simulink model "snc_sim"  (R2024b)
settings: Solver=VariableStepAuto  StartTime=0.0  StopTime=50  RelTol=1e-3
values from neighbouring files (symbols this model uses):
  GT = c2d(tf(wn^2,[1 2*wn*zeta wn^2]),Ts,'zoh')    [SNC.m]
  model = tf(bj_best.B*(K/y_model(end)),bj_best.F,Ts,'Variable','z^-1')    [SNC.m]
  R = x(nSint+2:end)'    [SNC.m]
  S = S.Numerator{1}    [SNC.m]
  T = P/sum(B)    [SNC.m]
  Ts = 0.3    [SNC.m]
settings Model: Creator=mihne  LastModifiedBy=Mihnea

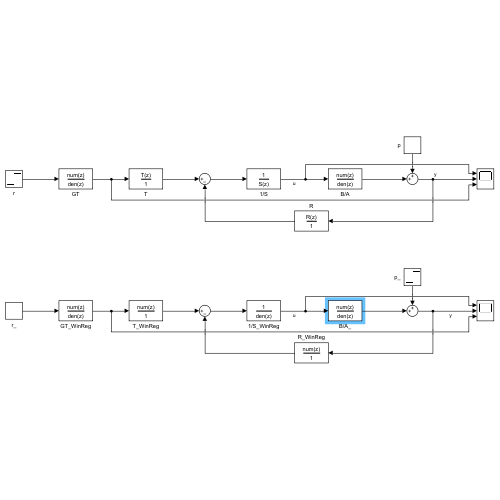
[thumbnail: Simulink's stored preview of the top-level diagram]
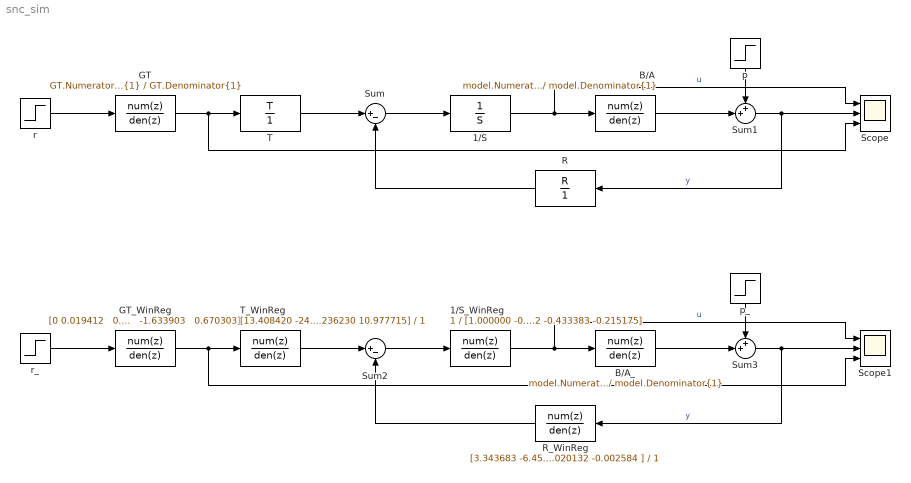
== system snc_sim ==
  1/S : DiscreteFilter  Numerator=1  Denominator=S
  1/S_WinReg : DiscreteFilter  Numerator=1  Denominator=[1.000000 -0.351442 -0.433383 -0.215175]
  B/A : DiscreteFilter  Numerator=model.Numerator{1}  Denominator=model.Denominator{1}
  B/A_ : DiscreteFilter  Numerator=model.Numerator{1}  Denominator=model.Denominator{1}
  GT : DiscreteFilter  Numerator=GT.Numerator{1}  Denominator=GT.Denominator{1}
  GT_WinReg : DiscreteFilter  Numerator="[0 0.019412   0.016988]"  Denominator="[1   -1.633903   0.670303]"
  R : DiscreteFilter  Numerator=R  Denominator=1
  R_WinReg : DiscreteFilter  Numerator=[3.343683 -6.451418 3.830355 -0.607159 0.016898 0.020132 -0.002584 ]  Denominator=1
  Scope : Scope  NumInputPorts=3
  Scope1 : Scope  NumInputPorts=3
  Sum : Sum  Inputs=|+-
  Sum1 : Sum  Inputs=++|
  Sum2 : Sum  Inputs=|+-
  Sum3 : Sum  Inputs=++|
  T : DiscreteFilter  Numerator=T  Denominator=1
  T_WinReg : DiscreteFilter  Numerator=[13.408420 -24.236230 10.977715]  Denominator=1
  p : Step  Time=25  After=33  SampleTime=Ts
  p_ : Step  Time=25  After=33  SampleTime=Ts
  r : Step  Time=0  After=132  SampleTime=Ts
  r_ : Step  Time=0  After=132  SampleTime=Ts
  wires:
  GT/1 -> Scope/3, T/1
  Sum/1 -> 1/S/1
  R/1 -> Sum/2
  1/S/1 -> Scope/1, B/A/1  "u"
  Sum1/1 -> R/1, Scope/2  "y"
  p/1 -> Sum1/1
  T/1 -> Sum/1
  B/A/1 -> Sum1/2
  R_WinReg/1 -> Sum2/2
  T_WinReg/1 -> Sum2/1
  p_/1 -> Sum3/1
  Sum2/1 -> 1/S_WinReg/1
  GT_WinReg/1 -> Scope1/3, T_WinReg/1
  1/S_WinReg/1 -> Scope1/1, B/A_/1  "u"
  r/1 -> GT/1
  B/A_/1 -> Sum3/2
  Sum3/1 -> R_WinReg/1, Scope1/2  "y"
  r_/1 -> GT_WinReg/1
